simulink model "JSimResultsModel1"  (R2021a)
settings: Solver=VariableStepAuto  StartTime=0.0  StopTime=50  RelTol=1e-3
values from neighbouring files (symbols this model uses):
  A = obj.networkMatrices.A    [Network.m]    (also in Subsystem.m = obj.A{obj.index}; jPaperData1.mat = [7.21225729966 1.39049686205 0 0 -0.282509513675 -0.19440187; jPaperData2.mat = [1.59283418225 -1.98990334273 -0.0774022354425 0.03883188575; paperData.mat = [-0.897343897753 -1.03363634124 0 0 0 0 -1.03363634124 -1.19)
  AcStab =     [jPaperData1.mat]    (also in jPaperData2.mat = [-4.66639923531 0.0224905641012 0.183856829633 -0.0600919958)
  B = obj.networkMatrices.B    [Network.m]    (also in Subsystem.m = obj.B{obj.index}; jPaperData1.mat = [0.133289291835 -2.25582289472 0 0 0 0 0 0 0 0 0 0 ... (50 e; jPaperData2.mat = [0.884783010265 -0.0578061269532 0 0 0 0 0 0 0 0 0 0 ... (50; paperData.mat = [-0.767652209467 0.0479827696564 0 0 0 0 0 0 0 0.69770450426)
  BcStab =     [jPaperData1.mat]    (also in jPaperData2.mat = [4.69331758427 -3.97574466957 -0.18243601768 0.0596281142245)
  C = obj.networkMatrices.C    [Network.m]    (also in Subsystem.m = {}; jPaperData1.mat = [-0.398868811937 0 0 0 0 0.199769403633 0 0 0 0 0 0 ... (50 ; jPaperData2.mat = [-2.29277321488 0 0 0 0 1.99520966434 0 0 0 0 0 0.4731154890; paperData.mat = [-0.192732954692 0 0 0.794595441386 0 0 0 1.44304729411 0 0 )
  CcStab =     [jPaperData1.mat]    (also in jPaperData2.mat = [3.40584102634 0.0670370876354 0 -0.466213574125 0.023320064)
  D = obj.networkMatrices.D    [Network.m]    (also in Subsystem.m = {}; jPaperData1.mat = [0 0 0 0 0 0 0 0 0 0 0 0 ... (25 elements, 5x5)]; jPaperData2.mat = [0 0 0 0 0 0 0 0 0 0 0 0 ... (25 elements, 5x5)]; paperData.mat = [0  0  0; 0  0  0; 0  0  0])
  DcStab =     [jPaperData1.mat]    (also in jPaperData2.mat = [-0.559949680356 -0.0227155093389 0 0.0369895329508 0.048553)
  E = obj.networkMatrices.E    [Network.m]    (also in Subsystem.m = {}; jPaperData1.mat = [0.013736298283 0.0126277412194 0 0 0 -0.00335268402912 0 0.; jPaperData2.mat = [-0.000849733283809 -0.00431479261265 0.00356522747973 0.001; paperData.mat = [0 0.622727541957 0 0 0 0 -0.10315996141 -0.125734072536 0 -)
  F = obj.networkMatrices.F    [Network.m]    (also in Subsystem.m = {}; jPaperData1.mat = [0 0 0 0 0 0 0.00667542601126 0 0 0 0 0 ... (25 elements, 5x; jPaperData2.mat = [0 0 0 0 0 0 0 0 0 0 0 0 ... (25 elements, 5x5)]; paperData.mat = [0.160906008337  0  0; 0  0.0149076612258  0; 0  0  0])
  G = obj.networkMatrices.G    [Network.m]    (also in Subsystem.m = {}; jPaperData1.mat = [1 0 0 0 0 1 0 0 0 0 0 1 ... (50 elements, 5x10)]; jPaperData2.mat = [1 0 0 0 0 1 0 0 0 0 0 1 ... (50 elements, 5x10)])
  H = obj.networkMatrices.H    [Network.m]    (also in Subsystem.m = {}; jPaperData1.mat = [1 0 0 0 0 0 1 0 0 0 0 0 ... (25 elements, 5x5)]; jPaperData2.mat = [1 0 0 0 0 0 1 0 0 0 0 0 ... (25 elements, 5x5)])
  J = obj.networkMatrices.J    [Network.m]    (also in Subsystem.m = {}; jPaperData1.mat = [1 0 0 0 0 0 1 0 0 0 0 0 ... (25 elements, 5x5)]; jPaperData2.mat = [1 0 0 0 0 0 1 0 0 0 0 0 ... (25 elements, 5x5)])
  KStab =     [jPaperData1.mat]    (also in jPaperData2.mat = [-4.86369493868 -0.00198336219621 0 -0.960462012264 -0.04588)
  LStab =     [jPaperData1.mat]    (also in jPaperData2.mat = [-2.23296914639 -0.236331029549 0.0275982481338 -0.070133150)
  n = size(A,1)    [Network.m]    (also in Subsystem.m = obj.dim_n; jPaperData1.mat = 10; jPaperData2.mat = 10; temp1.m)
libraries: simulink x1
settings Model: Creator=Shirantha Welikala  LastModifiedBy=Shirantha Welikala

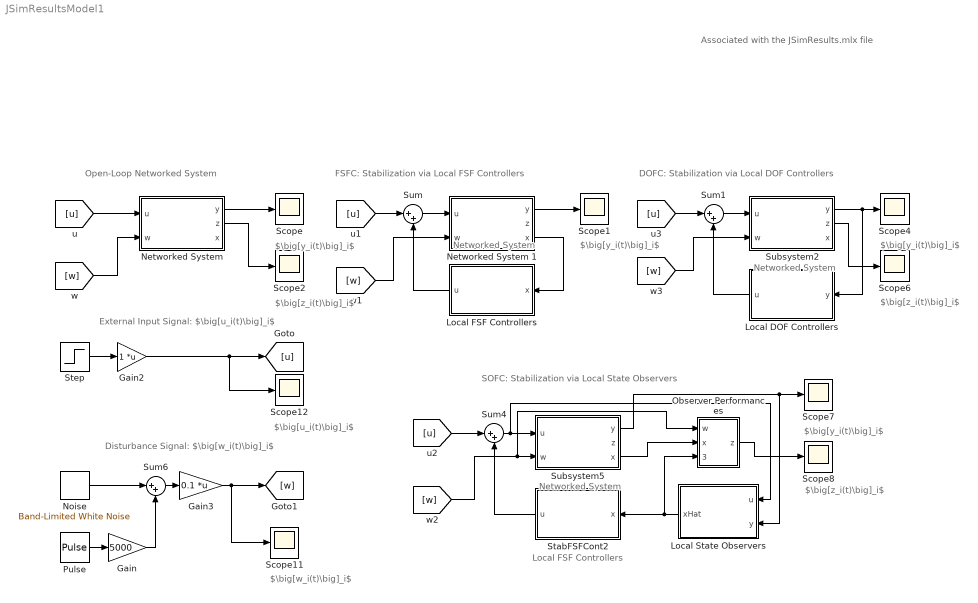
== system JSimResultsModel1 ==
  note: $\big[y_i(t)\big]_i$
  note: Local FSF Controllers
  note: Networked System
  note: External Input Signal: $\big[u_i(t)\big]_i$
  note: Associated with the JSimResults.mlx file
  note: Open-Loop Networked System
  note: FSFC: Stabilization via Local FSF Controllers
  note: DOFC: Stabilization via Local DOF Controllers
  note: SOFC: Stabilization via Local State Observers
  note: Disturbance Signal: $\big[w_i(t)\big]_i$
  note: Networked System
  note: Networked System
  note: $\big[y_i(t)\big]_i$
  note: $\big[y_i(t)\big]_i$
  note: $\big[z_i(t)\big]_i$
  note: $\big[z_i(t)\big]_i$
  note: $\big[y_i(t)\big]_i$
  note: $\big[w_i(t)\big]_i$
  note: $\big[u_i(t)\big]_i$
  note: $\big[z_i(t)\big]_i$
  Gain : Gain  Gain=5000
  Gain2 : Gain  Multiplication=Matrix(K*u)
  Gain3 : Gain  Gain=0.1  Multiplication=Matrix(K*u)
  Local DOF Controllers : Subsystem
  Local FSF Controllers : Subsystem
  Local State Observers : Subsystem
  Networked System : Subsystem
  Networked System 1 : Subsystem
  Noise : simulink/Sources/Band-Limited White Noise  Cov=[1]  Ts=0.01  seed=[23341]
  Observer Performances : Subsystem
  Pulse : DiscretePulseGenerator  PulseType=Time based  Period=10  PhaseDelay=5
  Scope{,1..2,4,6..8,11..12} (9 alike) : Scope
  StabFSFCont2 : Subsystem
  Step : Step  Time=5  Before=1  After=0  SampleTime=0
  Subsystem2 : Subsystem
  Subsystem5 : Subsystem
  Sum{,1,4,6} (4 alike) : Sum  Inputs=|++
  wires:
  Networked System/1(y) -> Scope/1
  [u] -> Networked System/1(u)
  Networked System 1/1(y) -> Scope1/1
  Networked System 1/3(x) -> Local FSF Controllers/1(x)
  [u] -> Sum/1
  Sum/1 -> Networked System 1/1(u)
  Local DOF Controllers/1(u) -> Sum1/2
  Subsystem2/1(y) -> Scope4/1, Local DOF Controllers/1(y)
  Sum1/1 -> Subsystem2/1(u)
  [w] -> Networked System 1/2(w)
  [w] -> Networked System/2(w)
  Local FSF Controllers/1(u) -> Sum/2
  Subsystem2/2(z) -> Scope6/1
  Sum4/1 -> Subsystem5/1(u), Local State Observers/1(u)
  StabFSFCont2/1(u) -> Sum4/2
  Subsystem5/3(x) -> Observer Performances/2(x)
  Subsystem5/1(y) -> Local State Observers/2(y), Scope7/1
  Observer Performances/1(z) -> Scope8/1
  Local State Observers/1(xHat) -> StabFSFCont2/1(x), Observer Performances/3(xHat)
  Noise/1 -> Sum6/1
  Sum6/1 -> Gain3/1
  Gain/1 -> Sum6/2
  Pulse/1 -> Gain/1
  Step/1 -> Gain2/1
  [u] -> Sum4/1
  [w] -> Subsystem5/2(w), Observer Performances/1(w)
  [u] -> Sum1/1
  [w] -> Subsystem2/2(w)
  Gain2/1 -> Scope12/1, [u]
  Gain3/1 -> Scope11/1, [w]
  Networked System/2(z) -> Scope2/1

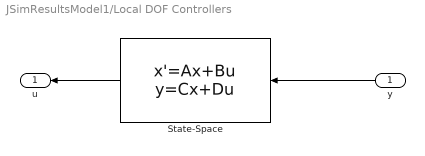
== system JSimResultsModel1/Local DOF Controllers ==
  y : Inport
  State-Space : StateSpace  A=AcStab  B=BcStab  C=CcStab  D=DcStab  InitialCondition=zeros(n,1)
  u : Outport
  wires:
  y/1 -> State-Space/1
  State-Space/1 -> u/1

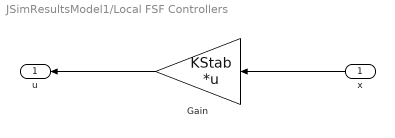
== system JSimResultsModel1/Local FSF Controllers ==
  x : Inport
  Gain : Gain  Gain=KStab  Multiplication=Matrix(K*u)
  u : Outport
  wires:
  x/1 -> Gain/1
  Gain/1 -> u/1

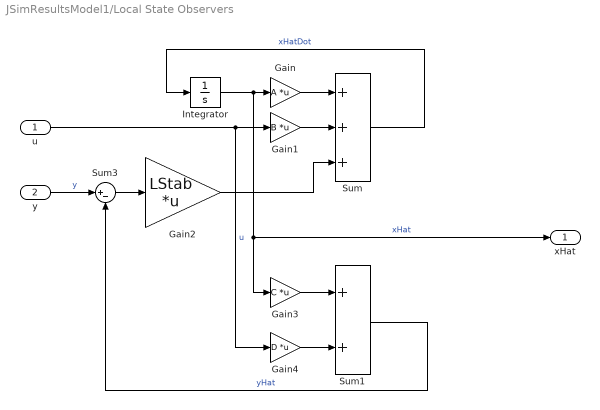
== system JSimResultsModel1/Local State Observers ==
  u : Inport
  y : Inport  Port=2
  Gain : Gain  Gain=A  Multiplication=Matrix(K*u)
  Gain1 : Gain  Gain=B  Multiplication=Matrix(K*u)
  Gain2 : Gain  Gain=LStab  Multiplication=Matrix(K*u)
  Gain3 : Gain  Gain=C  Multiplication=Matrix(K*u)
  Gain4 : Gain  Gain=D  Multiplication=Matrix(K*u)
  Integrator : Integrator  InitialCondition=zeros(n,1)
  Sum : Sum  Inputs=+++
  Sum1 : Sum
  Sum3 : Sum  Inputs=|+-
  xHat : Outport
  wires:
  Gain2/1 -> Sum/3
  Sum/1 -> Integrator/1  "xHatDot"
  Gain/1 -> Sum/1
  Gain1/1 -> Sum/2
  Integrator/1 -> Gain3/1, xHat/1, Gain/1  "xHat"
  u/1 -> Gain1/1, Gain4/1  "u"
  Gain4/1 -> Sum1/2
  Sum1/1 -> Sum3/2  "yHat"
  Gain3/1 -> Sum1/1
  y/1 -> Sum3/1  "y"
  Sum3/1 -> Gain2/1

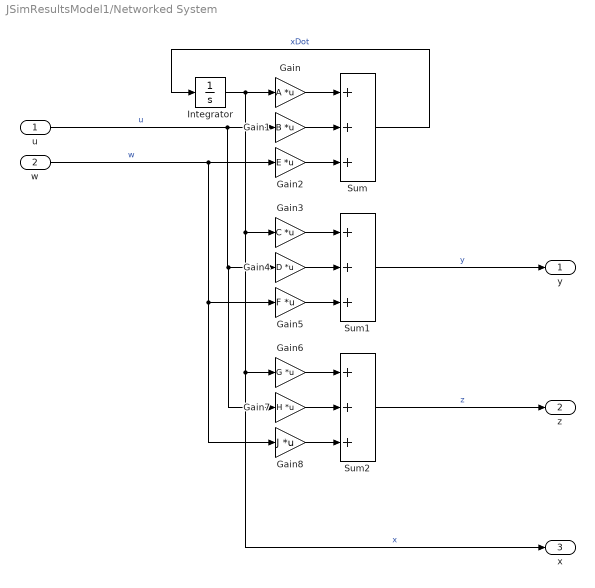
== system JSimResultsModel1/Networked System ==
  u : Inport
  w : Inport  Port=2
  Gain : Gain  Gain=A  Multiplication=Matrix(K*u)
  Gain1 : Gain  Gain=B  Multiplication=Matrix(K*u)
  Gain2 : Gain  Gain=E  Multiplication=Matrix(K*u)
  Gain3 : Gain  Gain=C  Multiplication=Matrix(K*u)
  Gain4 : Gain  Gain=D  Multiplication=Matrix(K*u)
  Gain5 : Gain  Gain=F  Multiplication=Matrix(K*u)
  Gain6 : Gain  Gain=G  Multiplication=Matrix(K*u)
  Gain7 : Gain  Gain=H  Multiplication=Matrix(K*u)
  Gain8 : Gain  Gain=J  Multiplication=Matrix(K*u)
  Integrator : Integrator  InitialCondition=10*ones(n,1)
  Sum : Sum  Inputs=+++
  Sum1 : Sum  Inputs=+++
  Sum2 : Sum  Inputs=+++
  y : Outport
  z : Outport  Port=2
  x : Outport  Port=3
  wires:
  u/1 -> Gain7/1, Gain4/1, Gain1/1  "u"
  Gain2/1 -> Sum/3
  w/1 -> Gain8/1, Gain5/1, Gain2/1  "w"
  Gain3/1 -> Sum1/1
  Sum/1 -> Integrator/1  "xDot"
  Gain5/1 -> Sum1/3
  Gain/1 -> Sum/1
  Gain1/1 -> Sum/2
  Gain4/1 -> Sum1/2
  Sum2/1 -> z/1  "z"
  Sum1/1 -> y/1  "y"
  Gain8/1 -> Sum2/3
  Gain6/1 -> Sum2/1
  Gain7/1 -> Sum2/2
  Integrator/1 -> x/1, Gain6/1, Gain3/1, Gain/1  "x"

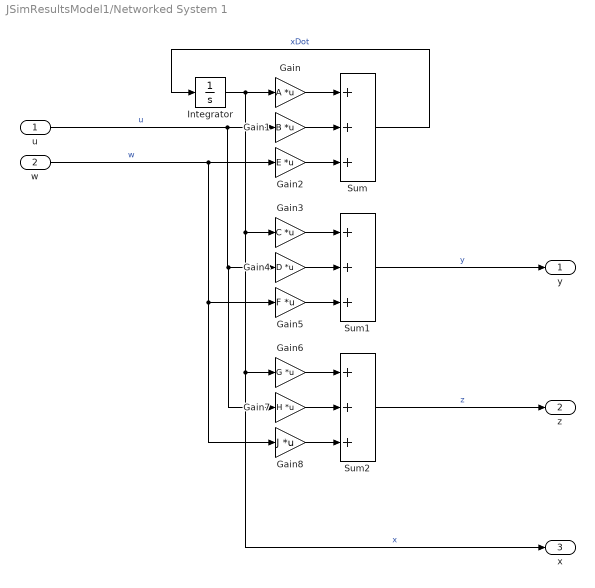
== system JSimResultsModel1/Networked System 1 ==
  u : Inport
  w : Inport  Port=2
  Gain : Gain  Gain=A  Multiplication=Matrix(K*u)
  Gain1 : Gain  Gain=B  Multiplication=Matrix(K*u)
  Gain2 : Gain  Gain=E  Multiplication=Matrix(K*u)
  Gain3 : Gain  Gain=C  Multiplication=Matrix(K*u)
  Gain4 : Gain  Gain=D  Multiplication=Matrix(K*u)
  Gain5 : Gain  Gain=F  Multiplication=Matrix(K*u)
  Gain6 : Gain  Gain=G  Multiplication=Matrix(K*u)
  Gain7 : Gain  Gain=H  Multiplication=Matrix(K*u)
  Gain8 : Gain  Gain=J  Multiplication=Matrix(K*u)
  Integrator : Integrator  InitialCondition=10*ones(n,1)
  Sum : Sum  Inputs=+++
  Sum1 : Sum  Inputs=+++
  Sum2 : Sum  Inputs=+++
  y : Outport
  z : Outport  Port=2
  x : Outport  Port=3
  wires:
  u/1 -> Gain7/1, Gain4/1, Gain1/1  "u"
  Gain2/1 -> Sum/3
  w/1 -> Gain8/1, Gain5/1, Gain2/1  "w"
  Gain3/1 -> Sum1/1
  Sum/1 -> Integrator/1  "xDot"
  Gain5/1 -> Sum1/3
  Gain/1 -> Sum/1
  Gain1/1 -> Sum/2
  Integrator/1 -> x/1, Gain6/1, Gain3/1, Gain/1  "x"
  Gain4/1 -> Sum1/2
  Sum2/1 -> z/1  "z"
  Sum1/1 -> y/1  "y"
  Gain8/1 -> Sum2/3
  Gain6/1 -> Sum2/1
  Gain7/1 -> Sum2/2

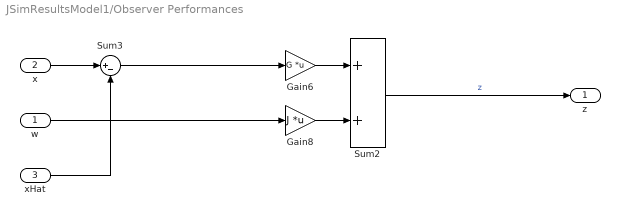
== system JSimResultsModel1/Observer Performances ==
  w : Inport
  x : Inport  Port=2
  xHat : Inport  Port=3
  Gain6 : Gain  Gain=G  Multiplication=Matrix(K*u)
  Gain8 : Gain  Gain=J  Multiplication=Matrix(K*u)
  Sum2 : Sum
  Sum3 : Sum  Inputs=|+-
  z : Outport
  wires:
  Gain8/1 -> Sum2/2
  Sum3/1 -> Gain6/1
  xHat/1 -> Sum3/2
  Gain6/1 -> Sum2/1
  Sum2/1 -> z/1  "z"
  w/1 -> Gain8/1
  x/1 -> Sum3/1

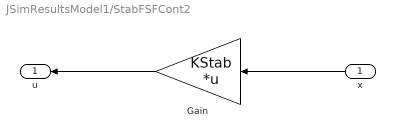
== system JSimResultsModel1/StabFSFCont2 ==
  x : Inport
  Gain : Gain  Gain=KStab  Multiplication=Matrix(K*u)
  u : Outport
  wires:
  x/1 -> Gain/1
  Gain/1 -> u/1

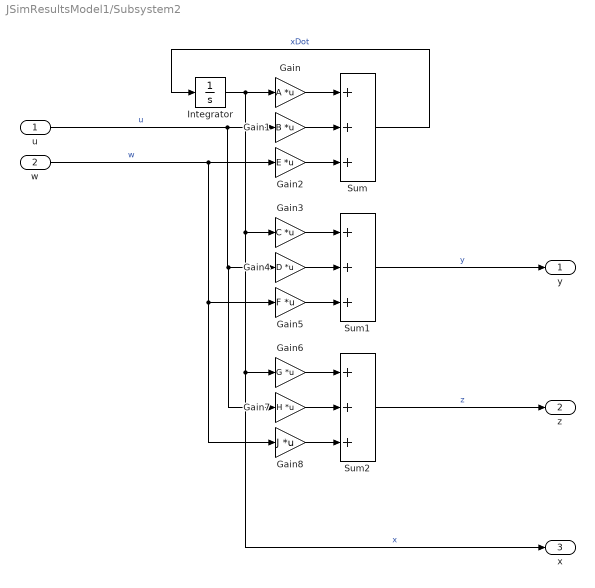
== system JSimResultsModel1/Subsystem2 ==
  u : Inport
  w : Inport  Port=2
  Gain : Gain  Gain=A  Multiplication=Matrix(K*u)
  Gain1 : Gain  Gain=B  Multiplication=Matrix(K*u)
  Gain2 : Gain  Gain=E  Multiplication=Matrix(K*u)
  Gain3 : Gain  Gain=C  Multiplication=Matrix(K*u)
  Gain4 : Gain  Gain=D  Multiplication=Matrix(K*u)
  Gain5 : Gain  Gain=F  Multiplication=Matrix(K*u)
  Gain6 : Gain  Gain=G  Multiplication=Matrix(K*u)
  Gain7 : Gain  Gain=H  Multiplication=Matrix(K*u)
  Gain8 : Gain  Gain=J  Multiplication=Matrix(K*u)
  Integrator : Integrator  InitialCondition=10*ones(n,1)
  Sum : Sum  Inputs=+++
  Sum1 : Sum  Inputs=+++
  Sum2 : Sum  Inputs=+++
  y : Outport
  z : Outport  Port=2
  x : Outport  Port=3
  wires:
  u/1 -> Gain7/1, Gain4/1, Gain1/1  "u"
  Gain2/1 -> Sum/3
  w/1 -> Gain8/1, Gain5/1, Gain2/1  "w"
  Gain3/1 -> Sum1/1
  Sum/1 -> Integrator/1  "xDot"
  Gain5/1 -> Sum1/3
  Gain/1 -> Sum/1
  Gain1/1 -> Sum/2
  Integrator/1 -> x/1, Gain6/1, Gain3/1, Gain/1  "x"
  Gain4/1 -> Sum1/2
  Sum2/1 -> z/1  "z"
  Sum1/1 -> y/1  "y"
  Gain8/1 -> Sum2/3
  Gain6/1 -> Sum2/1
  Gain7/1 -> Sum2/2

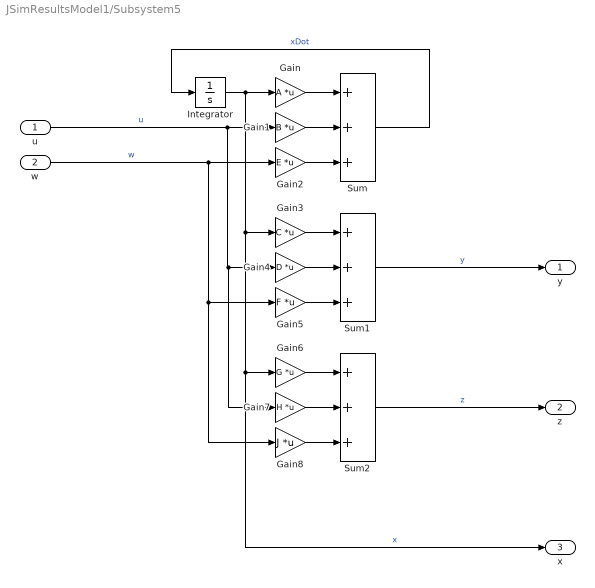
== system JSimResultsModel1/Subsystem5 ==
  u : Inport
  w : Inport  Port=2
  Gain : Gain  Gain=A  Multiplication=Matrix(K*u)
  Gain1 : Gain  Gain=B  Multiplication=Matrix(K*u)
  Gain2 : Gain  Gain=E  Multiplication=Matrix(K*u)
  Gain3 : Gain  Gain=C  Multiplication=Matrix(K*u)
  Gain4 : Gain  Gain=D  Multiplication=Matrix(K*u)
  Gain5 : Gain  Gain=F  Multiplication=Matrix(K*u)
  Gain6 : Gain  Gain=G  Multiplication=Matrix(K*u)
  Gain7 : Gain  Gain=H  Multiplication=Matrix(K*u)
  Gain8 : Gain  Gain=J  Multiplication=Matrix(K*u)
  Integrator : Integrator  InitialCondition=10*ones(n,1)
  Sum : Sum  Inputs=+++
  Sum1 : Sum  Inputs=+++
  Sum2 : Sum  Inputs=+++
  y : Outport
  z : Outport  Port=2
  x : Outport  Port=3
  wires:
  u/1 -> Gain7/1, Gain4/1, Gain1/1  "u"
  Gain2/1 -> Sum/3
  w/1 -> Gain8/1, Gain5/1, Gain2/1  "w"
  Gain3/1 -> Sum1/1
  Sum/1 -> Integrator/1  "xDot"
  Gain5/1 -> Sum1/3
  Gain/1 -> Sum/1
  Gain1/1 -> Sum/2
  Integrator/1 -> x/1, Gain6/1, Gain3/1, Gain/1  "x"
  Gain4/1 -> Sum1/2
  Sum2/1 -> z/1  "z"
  Sum1/1 -> y/1  "y"
  Gain8/1 -> Sum2/3
  Gain6/1 -> Sum2/1
  Gain7/1 -> Sum2/2
